simulink model "model"  (R2023b)
settings: Solver=VariableStepAuto  StartTime=0.0  StopTime=10.0  RelTol=1e-3
undefined symbols (not defined in the file): DiscIntNeverNeededParam, Newton, Raphson
libraries: simulink x77, slpidlib x18
(part 1 of 3)
settings Model: Creator=OSCAR4  LastModifiedBy=OSCAR4

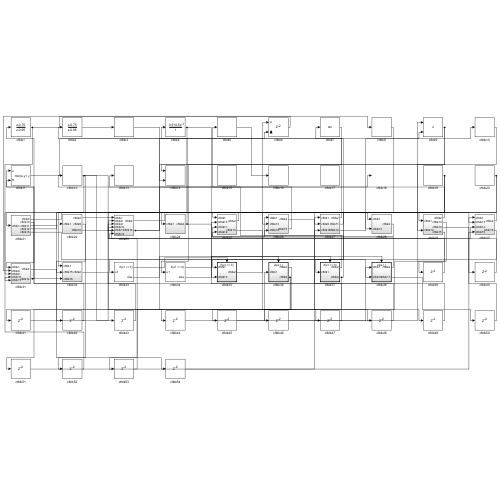
[thumbnail: Simulink's stored preview of the top-level diagram]
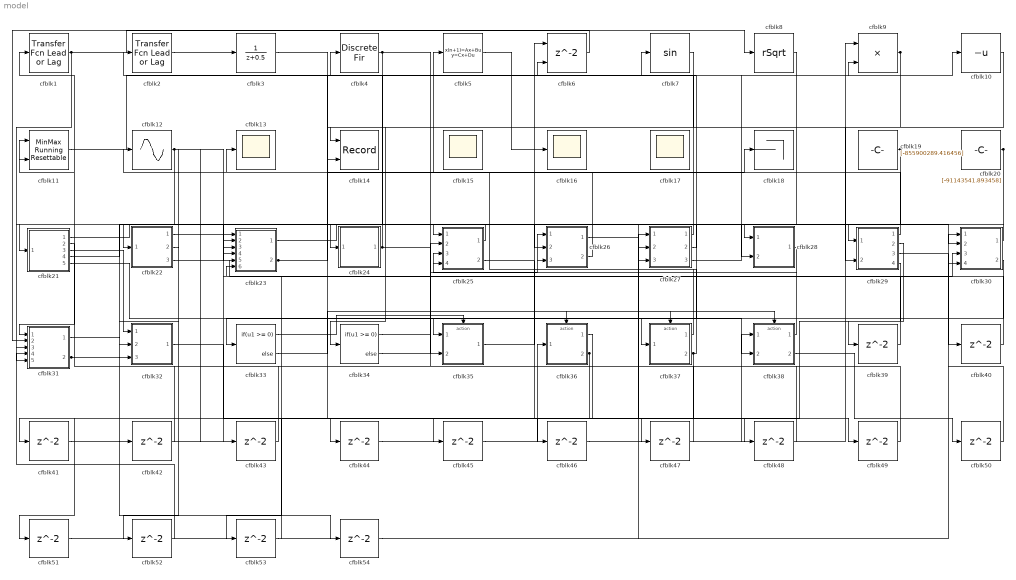
== system model ==
  cfblk1 : simulink/Discrete/Transfer Fcn Lead or Lag  PoleZ=0.95  ZeroZ=0.75  ICPrevOutput=0.0  ICPrevInput=0.0  DoSatur=off
  cfblk10 : UnaryMinus
  cfblk11 : simulink/Math Operations/MinMax Running Resettable  Function=min  vinit=0.0
  cfblk12 : Sin  TimeSource=Use external signal  SampleTime=0
  cfblk{13,15..17} (4 alike) : Scope
      cfblk15 settings: Floating=on
      cfblk17 settings: Floating=on
  cfblk14 : Record  FileSettingsInternal="{\"entries\":[{\"content\":{\"excelSettings\":{\"content\":{},\"type\":\"Streamout.ExcelSettings\"}},\"type\":\"Streamout.FileSettingStorage\",\"uuid\":\"\"}],\"packageUris\":[\"http:\\/\\/schema.mathworks.com\\/mf0\\/streamout_blocks\\/R2020a\"],\"version\":\"1.0\"}"  Layout=[1 1]  SignalsInternal="{\"entries\":[{\"content\":{\"signals\":[{\"content\":{\"blockPath\":[],\"dimensions\":[1],\"domain\":\"\",\"lineColor\":\"#a2142f\",\"plots\":[1],\"port\":1,\"signalID\":8231,\"signalName\":\"XY Graph:1\"},\"type\":\"RecordBlkView.Signal\",\"uuid\":\"\"},{\"content\":{\"blockPath\":[],\"dimensions\":[1],\"domain\":\"\",\"lineColor\":\"#139fff\",\"plots\":[1],\"port\":2,\"signalID\":8234,\"signalName\":\"XY Graph:2\"},\"type\":\"RecordBlkView.Signal\",\"uuid\":\"\"}]},\"type\":\"RecordBlkView.InputSignals\",\"uuid\":\"\"}],\"packageUris\":[\"http:\\/\\/schema.mathworks.com\\/mf0\\/streamout_blocks\\/R2020a\"],\"version\":\"1.0\"}"  VisualizationBindings="{\"xyplotplugin\":{\"info\":[{\"series\":[{\"bindingParametersList\":[{\"parameter\":\"X-Axis\",\"signalID\":8231,\"signalName\":\"XY Graph:1\"},{\"parameter\":\"Y-Axis\",\"signalID\":8234,\"signalName\":\"XY Graph:2\"}],\"seriesID\":32873}],\"subplotID\":1}]}}"  CompatibilityTag=XY
  cfblk18 : Terminator
  cfblk19 : Constant  Value=[-855900289.416456]  SampleTime=1
  cfblk2 : simulink/Discrete/Transfer Fcn Lead or Lag  PoleZ=0.95  ZeroZ=0.75  ICPrevOutput=0.0  ICPrevInput=0.0  DoSatur=off
  cfblk20 : Constant  Value=[-91143541.893458]  SampleTime=1
  cfblk21 : Subsystem
  cfblk22 : Subsystem
  cfblk23 : Subsystem
  cfblk24 : Subsystem
  cfblk25 : Subsystem
  cfblk26 : Subsystem
  cfblk27 : Subsystem
  cfblk28 : Subsystem
  cfblk29 : Subsystem
  cfblk3 : DiscreteTransferFcn  SampleTime=1
  cfblk30 : Subsystem
  cfblk31 : Subsystem
  cfblk32 : Subsystem
  cfblk33 : If  IfExpression=u1 >= 0  SampleTime=1
  cfblk34 : If  IfExpression=u1 >= 0  SampleTime=1
  cfblk35 : Subsystem  TreatAsAtomicUnit=on
  cfblk36 : Subsystem  TreatAsAtomicUnit=on
  cfblk37 : Subsystem  TreatAsAtomicUnit=on
  cfblk38 : Subsystem  TreatAsAtomicUnit=on
  cfblk{39..54} (16 alike) : Delay  SampleTime=1
  cfblk4 : DiscreteFir  SampleTime=1
  cfblk5 : DiscreteStateSpace
  cfblk6 : Delay  ShowEnablePort=on  SampleTime=1
      settings: InputPortMap=u0,e6
  cfblk7 : Trigonometry
  cfblk8 : Sqrt  Operator=rSqrt  AlgorithmType=Newton-Raphson
  cfblk9 : Product
  wires:
  cfblk21/1(cfblk2) -> cfblk25/1(cfblk1)
  cfblk21/2(cfblk10) -> cfblk31/1(cfblk1)
  cfblk5/1 -> cfblk16/1
  cfblk27/1(cfblk2) -> cfblk7/1
  cfblk19/1 -> cfblk33/1, cfblk37/1(cfblk1), cfblk35/2(cfblk13)
  cfblk20/1 -> cfblk21/1(cfblk1), cfblk31/3(cfblk9)
  cfblk29/1(cfblk2) -> cfblk5/1
  cfblk7/1 -> cfblk14/1
  cfblk6/1 -> cfblk31/2(cfblk8)
  cfblk31/2(cfblk12) -> cfblk11/1, cfblk54/1
  cfblk9/1 -> cfblk14/2, cfblk34/1
  cfblk2/1 -> cfblk3/1
  cfblk25/1(cfblk2) -> cfblk24/1(cfblk1)
  cfblk1/1 -> cfblk8/1, cfblk31/5(cfblk11)
  cfblk12/1 -> cfblk32/3(cfblk16), cfblk26/2(cfblk13), cfblk43/1, cfblk52/1
  cfblk30/1(cfblk2) -> cfblk29/1(cfblk1)
  cfblk24/1(cfblk2) -> cfblk2/1, cfblk26/3(cfblk14)
  cfblk11/1 -> cfblk9/2
  cfblk38/1(cfblk2) -> cfblk25/3(cfblk11)
  cfblk28/1(cfblk2) -> cfblk25/4(cfblk12)
  cfblk36/2(cfblk9) -> cfblk46/1, cfblk51/1
  cfblk37/1(cfblk2) -> cfblk12/1
  cfblk21/3(cfblk11) -> cfblk32/1(cfblk1)
  cfblk35/1(cfblk2) -> cfblk6/1
  cfblk10/1 -> cfblk29/2(cfblk12)
  cfblk4/1 -> cfblk22/1(cfblk1), cfblk28/2(cfblk13)
  cfblk30/2(cfblk16) -> cfblk35/1(cfblk1)
  cfblk26/2(cfblk15) -> cfblk13/1
  cfblk27/2(cfblk11) -> cfblk4/1
  cfblk37/2(cfblk8) -> cfblk26/1(cfblk1), cfblk53/1
  cfblk23/1(cfblk2) -> cfblk27/2(cfblk9)
  cfblk22/1(cfblk2) -> cfblk30/2(cfblk13)
  cfblk21/4(cfblk12) -> cfblk28/1(cfblk1)
  cfblk23/2(cfblk13) -> cfblk18/1, cfblk6/2
  cfblk21/5(cfblk13) -> cfblk38/2(cfblk16)
  cfblk22/2(cfblk9) -> cfblk32/2(cfblk15)
  cfblk22/3(cfblk10) -> cfblk30/3(cfblk14)
  cfblk27/3(cfblk12) -> cfblk10/1
  cfblk8/1 -> cfblk23/5(cfblk11)
  cfblk33/1 -> cfblk35/Action
  cfblk33/2 -> cfblk36/Action
  cfblk34/1 -> cfblk37/Action
  cfblk34/2 -> cfblk38/Action
  cfblk29/2(cfblk13) -> cfblk39/1
  cfblk39/1 -> cfblk23/1(cfblk1)
  cfblk29/3(cfblk14) -> cfblk40/1
  cfblk40/1 -> cfblk23/2(cfblk8)
  cfblk29/4(cfblk15) -> cfblk41/1
  cfblk41/1 -> cfblk23/4(cfblk10)
  cfblk31/1(cfblk2) -> cfblk42/1
  cfblk42/1 -> cfblk1/1
  cfblk43/1 -> cfblk11/2
  cfblk32/1(cfblk2) -> cfblk44/1
  cfblk44/1 -> cfblk36/1(cfblk1)
  cfblk36/1(cfblk2) -> cfblk45/1
  cfblk45/1 -> cfblk9/1
  cfblk46/1 -> cfblk38/1(cfblk1)
  cfblk3/1 -> cfblk47/1
  cfblk47/1 -> cfblk27/1(cfblk1)
  cfblk26/1(cfblk2) -> cfblk48/1
  cfblk48/1 -> cfblk25/2(cfblk10)
  cfblk25/2(cfblk13) -> cfblk49/1
  cfblk49/1 -> cfblk23/3(cfblk9)
  cfblk38/2(cfblk17) -> cfblk50/1
  cfblk50/1 -> cfblk30/1(cfblk1)
  cfblk51/1 -> cfblk27/3(cfblk10)
  cfblk52/1 -> cfblk31/4(cfblk10)
  cfblk53/1 -> cfblk23/6(cfblk12)
  cfblk54/1 -> cfblk30/4(cfblk15)

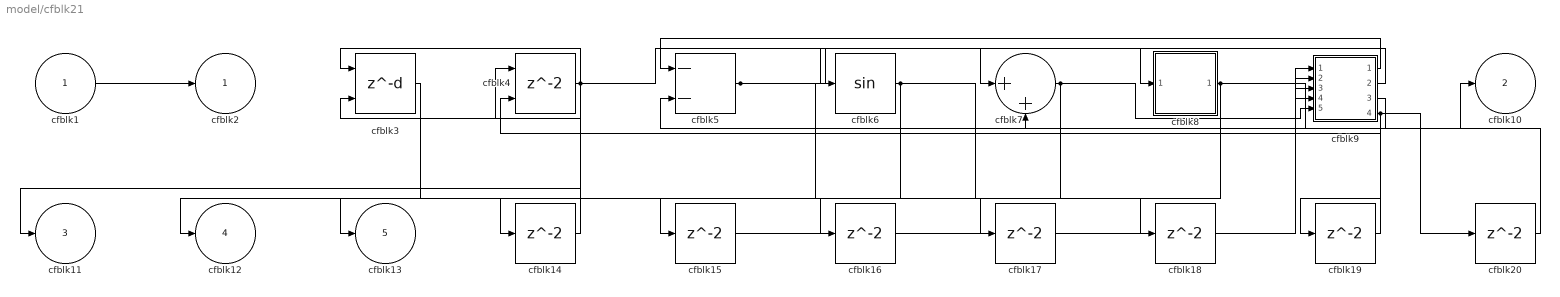
== system model/cfblk21 ==
  cfblk1 : Inport
  cfblk{14..20} (7 alike) : Delay  SampleTime=1
  cfblk3 : Delay  DelayLengthSource=Input port  SampleTime=1
      settings: InputPortMap=u0,p1
  cfblk4 : Delay  ShowEnablePort=on  SampleTime=1
      settings: InputPortMap=u0,e6
  cfblk5 : Sum  Inputs=--
  cfblk6 : Trigonometry
  cfblk7 : Sum  Inputs=|++
  cfblk8 : Subsystem
  cfblk9 : Subsystem
  cfblk2 : Outport
  cfblk10 : Outport  Port=2
  cfblk11 : Outport  Port=3
  cfblk12 : Outport  Port=4
  cfblk13 : Outport  Port=5
  wires:
  cfblk6/1 -> cfblk13/1, cfblk18/1
  cfblk1/1 -> cfblk2/1
  cfblk5/1 -> cfblk8/1(cfblk1), cfblk17/1
  cfblk9/1(cfblk2) -> cfblk5/1
  cfblk4/1 -> cfblk11/1, cfblk3/1, cfblk3/2, cfblk7/1
  cfblk9/2(cfblk15) -> cfblk6/1
  cfblk8/1(cfblk2) -> cfblk10/1, cfblk15/1, cfblk16/1
  cfblk7/1 -> cfblk9/5(cfblk14), cfblk14/1
  cfblk3/1 -> cfblk12/1
  cfblk9/3(cfblk16) -> cfblk5/2
  cfblk9/4(cfblk17) -> cfblk19/1, cfblk20/1
  cfblk14/1 -> cfblk4/1
  cfblk15/1 -> cfblk9/3(cfblk12)
  cfblk16/1 -> cfblk9/4(cfblk13)
  cfblk17/1 -> cfblk9/2(cfblk11)
  cfblk18/1 -> cfblk9/1(cfblk1)
  cfblk19/1 -> cfblk4/2
  cfblk20/1 -> cfblk7/2

== system model/cfblk22 ==
  cfblk1 : Inport
  cfblk{3,11..17} (8 alike) : Delay  SampleTime=1
  cfblk4 : Subsystem
  cfblk5 : Subsystem
  cfblk6 : Subsystem
  cfblk7 : Subsystem
  cfblk8 : Subsystem
  cfblk2 : Outport
  cfblk9 : Outport  Port=2
  cfblk10 : Outport  Port=3
  wires:
  cfblk1/1 -> cfblk8/1(cfblk1)
  cfblk8/1(cfblk2) -> cfblk6/1(cfblk1)
  cfblk4/1(cfblk2) -> cfblk7/1(cfblk1)
  cfblk5/1(cfblk2) -> cfblk3/1
  cfblk3/1 -> cfblk10/1, cfblk4/2(cfblk13), cfblk4/3(cfblk14), cfblk16/1
  cfblk6/1(cfblk2) -> cfblk2/1
  cfblk8/2(cfblk10) -> cfblk5/1(cfblk1)
  cfblk8/3(cfblk11) -> cfblk5/2(cfblk11), cfblk9/1, cfblk4/5(cfblk16)
  cfblk6/2(cfblk9) -> cfblk5/3(cfblk12)
  cfblk5/3(cfblk16) -> cfblk7/2(cfblk9)
  cfblk7/3(cfblk11) -> cfblk13/1, cfblk14/1
  cfblk7/1(cfblk2) -> cfblk11/1
  cfblk11/1 -> cfblk6/4(cfblk8)
  cfblk7/2(cfblk10) -> cfblk12/1
  cfblk12/1 -> cfblk4/1(cfblk1)
  cfblk13/1 -> cfblk5/4(cfblk13)
  cfblk14/1 -> cfblk4/4(cfblk15)
  cfblk4/2(cfblk17) -> cfblk15/1
  cfblk15/1 -> cfblk6/2(cfblk6)
  cfblk16/1 -> cfblk5/5(cfblk14)
  cfblk5/2(cfblk15) -> cfblk17/1
  cfblk17/1 -> cfblk6/3(cfblk7)

== system model/cfblk23 ==
  cfblk1 : Inport
  cfblk8 : Inport  Port=2
  cfblk9 : Inport  Port=3
  cfblk10 : Inport  Port=4
  cfblk11 : Inport  Port=5
  cfblk12 : Inport  Port=6
  cfblk14 : Delay  SampleTime=1
  cfblk15 : Delay  SampleTime=1
  cfblk3 : Delay  ShowEnablePort=on  SampleTime=1
      settings: InputPortMap=u0,e6
  cfblk4 : DotProduct  OutDataTypeStr=Inherit: Inherit via internal rule
  cfblk5 : Subsystem
  cfblk6 : Subsystem
  cfblk7 : Subsystem
  cfblk2 : Outport
  cfblk13 : Outport  Port=2
  wires:
  cfblk4/1 -> cfblk7/1(cfblk1)
  cfblk8/1 -> cfblk5/1(cfblk1)
  cfblk6/2(cfblk10) -> cfblk5/2(cfblk6)
  cfblk12/1 -> cfblk3/2
  cfblk9/1 -> cfblk6/1(cfblk1)
  cfblk3/1 -> cfblk6/2(cfblk8)
  cfblk11/1 -> cfblk4/1
  cfblk7/1(cfblk2) -> cfblk6/3(cfblk9)
  cfblk7/2(cfblk13) -> cfblk2/1, cfblk15/1
  cfblk1/1 -> cfblk5/3(cfblk7)
  cfblk10/1 -> cfblk5/4(cfblk8)
  cfblk5/1(cfblk2) -> cfblk13/1
  cfblk6/1(cfblk2) -> cfblk14/1
  cfblk14/1 -> cfblk3/1
  cfblk15/1 -> cfblk4/2

== system model/cfblk24 ==
  cfblk1 : Inport
  cfblk10 : Delay  SampleTime=1
  cfblk3 : DiscreteFilter  SampleTime=1
  cfblk4 : DiscreteFir  SampleTime=1
  cfblk5 : DiscreteZeroPole  Poles=[0 0.5]  Gain=1
  cfblk6 : Delay  SampleTime=1
  cfblk7 : Constant  Value=[-62407145.955087]  SampleTime=1
  cfblk8 : Constant  Value=[-969597056.657864]  SampleTime=1
  cfblk9 : Constant  Value=[861290801.323652]  SampleTime=1
  cfblk2 : Outport
  wires:
  cfblk7/1 -> cfblk5/1
  cfblk1/1 -> cfblk3/1
  cfblk4/1 -> cfblk6/1
  cfblk5/1 -> cfblk2/1
  cfblk6/1 -> cfblk10/1
  cfblk10/1 -> cfblk4/1

== system model/cfblk25 ==
  cfblk1 : Inport
  cfblk10 : Inport  Port=2
  cfblk11 : Inport  Port=3
  cfblk12 : Inport  Port=4
  cfblk3 : DiscreteFir  SampleTime=1
  cfblk4 : simulink/Discrete/Difference  ICPrevInput=0.0  OutMin=[]  OutMax=[]  OutDataTypeStr=Inherit: Inherit via back propagation  OutDataType=fixdt(1, 16)  OutScaling=2^-10  DoSatur=off
  cfblk5 : Product
  cfblk6 : Sqrt
  cfblk7 : Constant  Value=[-116065568.757723]  SampleTime=1
  cfblk8 : Constant  Value=[768182998.999454]  SampleTime=1
  cfblk9 : Subsystem
  cfblk2 : Outport
  cfblk13 : Outport  Port=2
  wires:
  cfblk1/1 -> cfblk4/1
  cfblk8/1 -> cfblk3/1
  cfblk11/1 -> cfblk2/1
  cfblk10/1 -> cfblk9/1(cfblk1)
  cfblk7/1 -> cfblk13/1
  cfblk5/1 -> cfblk9/2(cfblk5)
  cfblk12/1 -> cfblk6/1
  cfblk6/1 -> cfblk5/1
  cfblk3/1 -> cfblk9/3(cfblk6)
  cfblk4/1 -> cfblk5/2

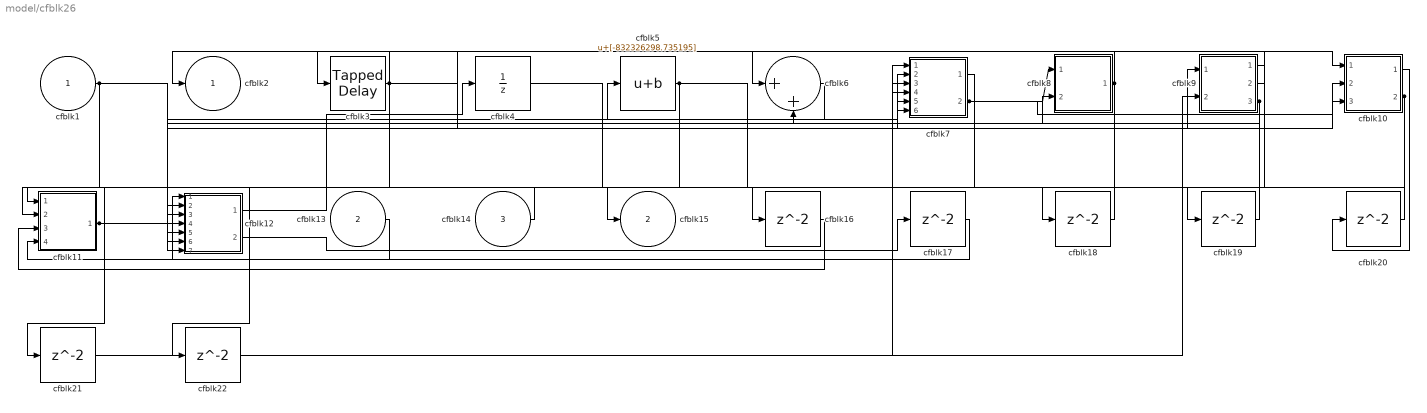
== system model/cfblk26 ==
  cfblk1 : Inport
  cfblk13 : Inport  Port=2
  cfblk14 : Inport  Port=3
  cfblk10 : Subsystem
  cfblk11 : Subsystem
  cfblk12 : Subsystem
  cfblk{16..22} (7 alike) : Delay  SampleTime=1
  cfblk3 : simulink/Discrete/Tapped Delay  vinit=0.0  samptime=-1  NumDelays=1  DelayOrder=Oldest  includeCurrent=off
  cfblk4 : UnitDelay  HasFrameUpgradeWarning=on
  cfblk5 : Bias  Bias=[-832326298.735195]  SaturateOnIntegerOverflow=off
  cfblk6 : Sum  Inputs=|++
  cfblk7 : Subsystem
  cfblk8 : Subsystem
  cfblk9 : Subsystem
  cfblk2 : Outport
  cfblk15 : Outport  Port=2
  wires:
  cfblk5/1 -> cfblk12/5(cfblk13), cfblk19/1
  cfblk1/1 -> cfblk11/1(cfblk1), cfblk7/6(cfblk11)
  cfblk9/1(cfblk2) -> cfblk15/1
  cfblk12/1(cfblk2) -> cfblk4/1
  cfblk13/1 -> cfblk12/1(cfblk1)
  cfblk6/1 -> cfblk5/1
  cfblk3/1 -> cfblk2/1, cfblk8/2(cfblk8), cfblk10/1(cfblk1), cfblk10/3(cfblk11), cfblk22/1
  cfblk14/1 -> cfblk12/2(cfblk10)
  cfblk9/2(cfblk13) -> cfblk3/1
  cfblk9/3(cfblk14) -> cfblk7/2(cfblk7), cfblk12/6(cfblk14)
  cfblk7/1(cfblk2) -> cfblk12/3(cfblk11)
  cfblk8/1(cfblk2) -> cfblk6/1, cfblk18/1
  cfblk10/2(cfblk12) -> cfblk12/4(cfblk12), cfblk12/7(cfblk15), cfblk21/1
  cfblk11/1(cfblk2) -> cfblk7/5(cfblk10), cfblk6/2, cfblk9/1(cfblk1)
  cfblk7/2(cfblk12) -> cfblk8/1(cfblk1), cfblk10/2(cfblk10)
  cfblk4/1 -> cfblk16/1
  cfblk16/1 -> cfblk11/3(cfblk9)
  cfblk12/2(cfblk16) -> cfblk17/1
  cfblk17/1 -> cfblk11/4(cfblk10)
  cfblk18/1 -> cfblk7/3(cfblk8)
  cfblk19/1 -> cfblk7/1(cfblk1)
  cfblk10/1(cfblk2) -> cfblk20/1
  cfblk20/1 -> cfblk11/2(cfblk8)
  cfblk21/1 -> cfblk7/4(cfblk9)
  cfblk22/1 -> cfblk9/2(cfblk12)

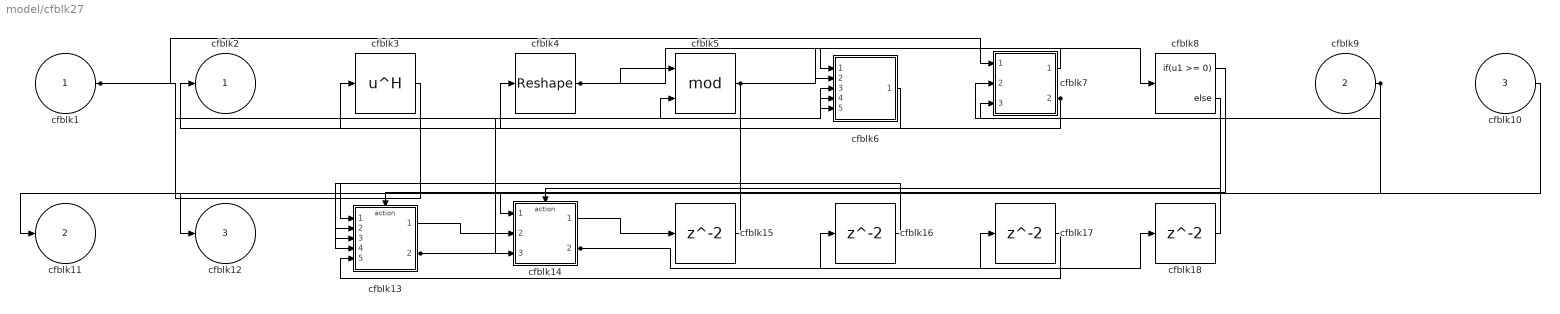
== system model/cfblk27 ==
  cfblk1 : Inport
  cfblk9 : Inport  Port=2
  cfblk10 : Inport  Port=3
  cfblk13 : Subsystem  TreatAsAtomicUnit=on
  cfblk14 : Subsystem  TreatAsAtomicUnit=on
  cfblk{15..18} (4 alike) : Delay  SampleTime=1
  cfblk3 : Math  Operator=hermitian
  cfblk4 : Reshape
  cfblk5 : Math  Operator=mod
  cfblk6 : Subsystem
  cfblk7 : Subsystem
  cfblk8 : If  IfExpression=u1 >= 0  SampleTime=1
  cfblk2 : Outport
  cfblk11 : Outport  Port=2
  cfblk12 : Outport  Port=3
  wires:
  cfblk4/1 -> cfblk6/1(cfblk1), cfblk5/1
  cfblk10/1 -> cfblk11/1
  cfblk9/1 -> cfblk14/1(cfblk1), cfblk14/3(cfblk14), cfblk7/3(cfblk12)
  cfblk6/1(cfblk2) -> cfblk2/1
  cfblk1/1 -> cfblk7/1(cfblk1), cfblk13/4(cfblk14), cfblk5/2
  cfblk14/2(cfblk15) -> cfblk16/1, cfblk17/1, cfblk18/1
  cfblk3/1 -> cfblk13/3(cfblk13)
  cfblk5/1 -> cfblk12/1, cfblk8/1
  cfblk7/1(cfblk2) -> cfblk6/2(cfblk8)
  cfblk13/1(cfblk2) -> cfblk14/2(cfblk13)
  cfblk7/2(cfblk13) -> cfblk3/1, cfblk4/1
  cfblk13/2(cfblk16) -> cfblk6/3(cfblk9), cfblk6/4(cfblk10), cfblk6/5(cfblk11)
  cfblk8/1 -> cfblk13/Action
  cfblk8/2 -> cfblk14/Action
  cfblk14/1(cfblk2) -> cfblk15/1
  cfblk15/1 -> cfblk13/1(cfblk1)
  cfblk16/1 -> cfblk13/2(cfblk12)
  cfblk17/1 -> cfblk13/5(cfblk15)
  cfblk18/1 -> cfblk7/2(cfblk11)

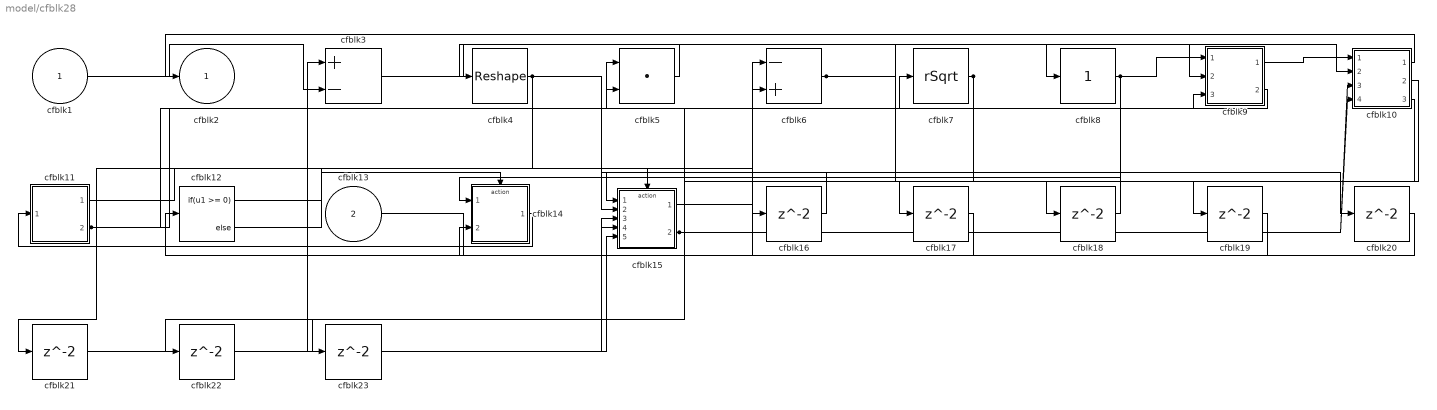
== system model/cfblk28 ==
  cfblk1 : Inport
  cfblk13 : Inport  Port=2
  cfblk10 : Subsystem
  cfblk11 : Subsystem
  cfblk12 : If  IfExpression=u1 >= 0  SampleTime=1
  cfblk14 : Subsystem  TreatAsAtomicUnit=on
  cfblk15 : Subsystem  TreatAsAtomicUnit=on
  cfblk{16..23} (8 alike) : Delay  SampleTime=1
  cfblk3 : Sum  Inputs=+-
  cfblk4 : Reshape
  cfblk5 : DotProduct  OutDataTypeStr=Inherit: Inherit via internal rule
  cfblk6 : Sum  Inputs=-+
  cfblk7 : Sqrt  Operator=rSqrt  AlgorithmType=Newton-Raphson
  cfblk8 : simulink/Math Operations/Slider Gain  gain=1  low=0  high=2
  cfblk9 : Subsystem
  cfblk2 : Outport
  wires:
  cfblk3/1 -> cfblk8/1
  cfblk13/1 -> cfblk6/1
  cfblk15/1(cfblk2) -> cfblk6/2
  cfblk8/1 -> cfblk14/1(cfblk1), cfblk9/1(cfblk1)
  cfblk11/2(cfblk11) -> cfblk7/1, cfblk9/3(cfblk11)
  cfblk7/1 -> cfblk22/1, cfblk23/1
  cfblk14/1(cfblk2) -> cfblk11/1(cfblk1)
  cfblk5/1 -> cfblk4/1
  cfblk9/1(cfblk2) -> cfblk10/1(cfblk1)
  cfblk15/2(cfblk15) -> cfblk5/1, cfblk10/3(cfblk14), cfblk10/4(cfblk15)
  cfblk6/1 -> cfblk10/2(cfblk13), cfblk9/2(cfblk10), cfblk19/1
  cfblk1/1 -> cfblk3/2
  cfblk9/2(cfblk12) -> cfblk5/2
  cfblk4/1 -> cfblk20/1, cfblk21/1
  cfblk10/1(cfblk2) -> cfblk2/1
  cfblk12/1 -> cfblk14/Action
  cfblk12/2 -> cfblk15/Action
  cfblk11/1(cfblk2) -> cfblk16/1
  cfblk16/1 -> cfblk15/1(cfblk1)
  cfblk10/2(cfblk16) -> cfblk17/1
  cfblk17/1 -> cfblk14/2(cfblk10)
  cfblk10/3(cfblk17) -> cfblk18/1
  cfblk18/1 -> cfblk15/2(cfblk11)
  cfblk19/1 -> cfblk15/4(cfblk13)
  cfblk20/1 -> cfblk12/1
  cfblk21/1 -> cfblk15/5(cfblk14)
  cfblk22/1 -> cfblk3/1
  cfblk23/1 -> cfblk15/3(cfblk12)

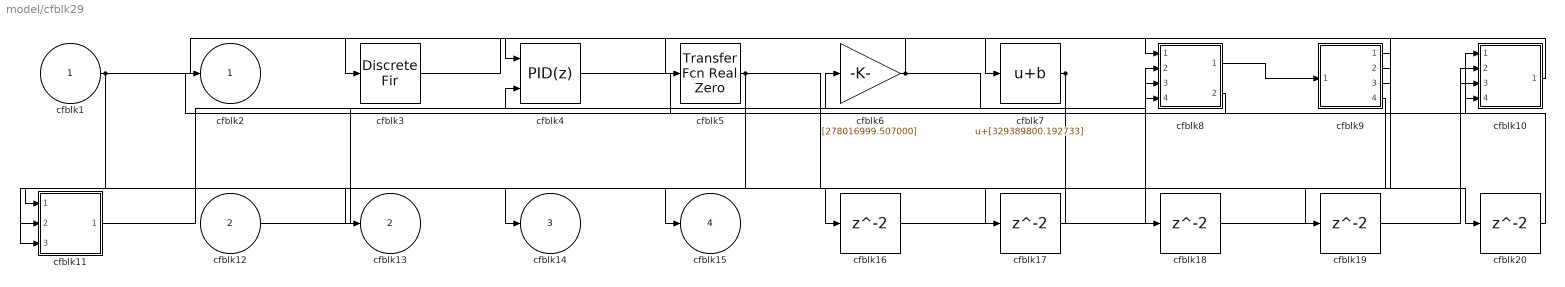
== system model/cfblk29 ==
  cfblk1 : Inport
  cfblk12 : Inport  Port=2
  cfblk10 : Subsystem
  cfblk11 : Subsystem
  cfblk{16..20} (5 alike) : Delay  SampleTime=1
  cfblk3 : DiscreteFir  SampleTime=1
  cfblk4 : slpidlib/PID Controller (2DOF)  Controller=PID  Form=Parallel  TimeDomain=Discrete-time  UseExternalTs=off  SampleTime=1  IntegratorMethod=Forward Euler  FilterMethod=Forward Euler  ControllerParametersSource=internal  P=1  I=1  UseKiTs=off  D=0  N=100  UseFilter=on  b=1  c=1  TunerSelectOption=Transfer Function Based (PID Tuner App)  InitialConditionSource=internal  InitialConditionForIntegrator=0  InitialConditionForFilter=0  DifferentiatorICPrevScaledInput=0  ExternalReset=none  TrackingMode=off  Kt=1  LimitOutput=off  SatLimitsSource=internal  UpperSaturationLimit=inf  LowerSaturationLimit=-inf  LinearizeAsGain=off  AntiWindupMode=none  Kb=1  LimitIntegrator=off  UpperIntegratorSaturationLimit=inf  LowerIntegratorSaturationLimit=-inf  POutMin=[]  POutMax=[]  IOutMin=[]  IOutMax=[]  DOutMin=[]  DOutMax=[]  NOutMin=[]  NOutMax=[]  bOutMin=[]  bOutMax=[]  cOutMin=[]  cOutMax=[]  SumOutMin=[]  SumOutMax=[]  SaturationOutMin=[]  SaturationOutMax=[]  PParamMin=[]  PParamMax=[]  IParamMin=[]  IParamMax=[]  DParamMin=[]  DParamMax=[]  NParamMin=[]  NParamMax=[]  bParamMin=[]  bParamMax=[]  cParamMin=[]  cParamMax=[]  KbParamMin=[]  KbParamMax=[]  KtParamMin=[]  KtParamMax=[]  KbOutMin=[]  KbOutMax=[]  KtOutMin=[]  KtOutMax=[]  IntegratorOutMin=[]  IntegratorOutMax=[]  FilterOutMin=[]  FilterOutMax=[]  SumI1OutMin=[]  SumI1OutMax=[]  SumI2OutMin=[]  SumI2OutMax=[]  SumI3OutMin=[]  SumI3OutMax=[]  SumI4OutMin=[]  SumI4OutMax=[]  SumDOutMin=[]  SumDOutMax=[]  Sum1OutMin=[]  Sum1OutMax=[]  Sum2OutMin=[]  Sum2OutMax=[]  Sum3OutMin=[]  Sum3OutMax=[]  DifferentiatorOutMin=[]  DifferentiatorOutMax=[]  FilterDiffOutCoefMin=[]  FilterDiffOutCoefMax=[]  ReciprocalOutMin=[]  ReciprocalOutMax=[]  SumDenOutMin=[]  SumDenOutMax=[]  SumNumOutMin=[]  SumNumOutMax=[]  DivideOutMin=[]  DivideOutMax=[]  UdiffTsProdOutMin=[]  UdiffTsProdOutMax=[]  NTsProdOutMin=[]  NTsProdOutMax=[]  UintegralTsProdOutMin=[]  UintegralTsProdOutMax=[]  UngainTsProdOutMin=[]  UngainTsProdOutMax=[]  ClampingZeroOutDataTypeStr=Inherit: Inherit via back propagation  ClampingZeroOutMin=[]  ClampingZeroOutMax=[]  FilterDenConstantOutDataTypeStr=Inherit: Inherit via back propagation  FilterDenConstantOutMin=[]  FilterDenConstantOutMax=[]  PCopyOutDataTypeStr=Inherit: Inherit via back propagation  PCopyOutMin=[]  PCopyOutMax=[]  NCopyOutDataTypeStr=Inherit: Inherit via back propagation  NCopyOutMin=[]  NCopyOutMax=[]  IntegratorContinuousStateAttributes=''  IntegratorStateMustResolveToSignalObject=off  IntegratorRTWStateStorageClass=Auto  FilterContinuousStateAttributes=''  FilterStateMustResolveToSignalObject=off  FilterRTWStateStorageClass=Auto  ParallelPVariant=InternalParameters  IdealPVariant=Disabled  IVariant=InternalParameters  DVariant=InternalParameters  bVariant=InternalParameters  cVariant=InternalParameters  IntegratorVariant=Discrete  SatVariant=Disabled  AWVariant=Passthrough  PCopyVariant=Disabled  TRVariant=Disabled  FdbkBlocksVariant=Forward  IdealPFdbkVariant=Disabled  SatFdbkVariant=Disabled  DerivativeFilterVariant=ForwardEulerFilter  NVariant=InternalParameters  NCopyVariant=Disabled  FilterICVariant=InternalICsFilter  IntegratorICVariant=InternalICs  ExternalResetVariant=Disabled  TRSumVariant=Passthrough  SumFdbkVariant=Disabled  SumVariant=Sum_PID  TsampFilterVariant=InternalTs  TsampNgainVariant=Passthrough  TsampIntegralVariant=Disabled_SignalSpec  ExternalSaturationOutDataTypeStr=Inherit: Same as second input
      settings: LibrarySourceBlock=simulink/Discrete/Discrete PID Controller (2DOF)
  cfblk5 : simulink/Discrete/Transfer Fcn Real Zero  ZeroZ=0.75  ICPrevInput=0.0  DoSatur=off
  cfblk6 : Gain  Gain=[278016999.507000]
  cfblk7 : Bias  Bias=[329389800.192733]  SaturateOnIntegerOverflow=off
  cfblk8 : Subsystem
  cfblk9 : Subsystem
  cfblk2 : Outport
  cfblk13 : Outport  Port=2
  cfblk14 : Outport  Port=3
  cfblk15 : Outport  Port=4
  wires:
  cfblk6/1 -> cfblk3/1, cfblk8/3(cfblk14)
  cfblk4/1 -> cfblk10/1(cfblk1)
  cfblk12/1 -> cfblk6/1
  cfblk10/1(cfblk2) -> cfblk5/1
  cfblk1/1 -> cfblk4/1, cfblk11/3(cfblk8)
  cfblk5/1 -> cfblk11/1(cfblk1), cfblk13/1, cfblk11/2(cfblk7), cfblk19/1, cfblk20/1
  cfblk8/1(cfblk2) -> cfblk9/1(cfblk1)
  cfblk8/2(cfblk16) -> cfblk2/1
  cfblk3/1 -> cfblk8/1(cfblk1)
  cfblk9/1(cfblk2) -> cfblk14/1
  cfblk11/1(cfblk2) -> cfblk8/2(cfblk13)
  cfblk9/2(cfblk12) -> cfblk7/1
  cfblk7/1 -> cfblk15/1, cfblk16/1
  cfblk16/1 -> cfblk8/4(cfblk15)
  cfblk9/3(cfblk13) -> cfblk17/1
  cfblk17/1 -> cfblk4/2
  cfblk9/4(cfblk14) -> cfblk18/1
  cfblk18/1 -> cfblk10/2(cfblk14)
  cfblk19/1 -> cfblk10/3(cfblk15)
  cfblk20/1 -> cfblk10/4(cfblk16)

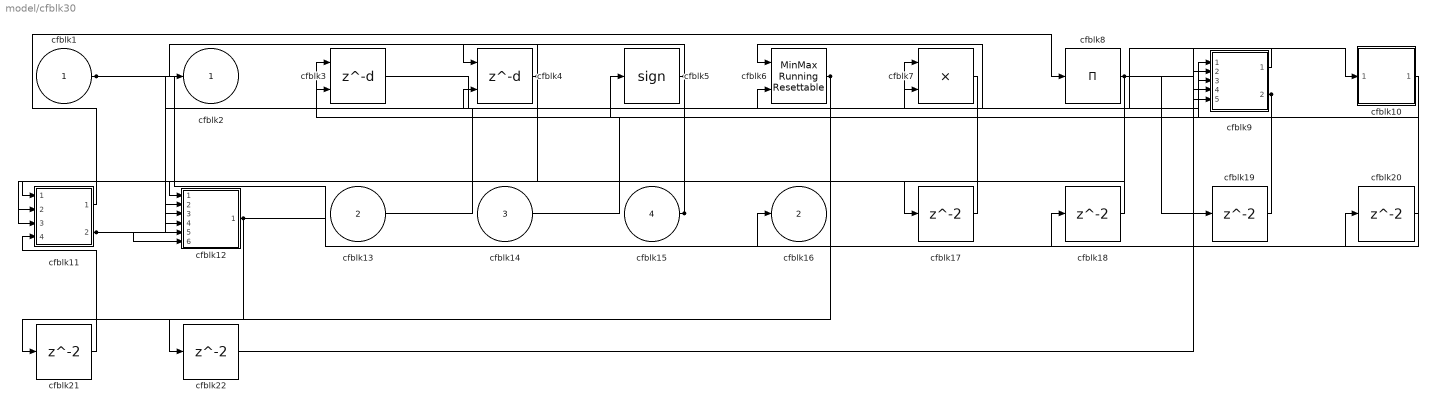
== system model/cfblk30 ==
  cfblk1 : Inport
  cfblk13 : Inport  Port=2
  cfblk14 : Inport  Port=3
  cfblk15 : Inport  Port=4
  cfblk10 : Subsystem
  cfblk11 : Subsystem
  cfblk12 : Subsystem
  cfblk{17..22} (6 alike) : Delay  SampleTime=1
  cfblk3 : Delay  DelayLengthSource=Input port  SampleTime=1
      settings: InputPortMap=u0,p1
  cfblk4 : Delay  DelayLengthSource=Input port  SampleTime=1
      settings: InputPortMap=u0,p1
  cfblk5 : Signum
  cfblk6 : simulink/Math Operations/MinMax Running Resettable  Function=min  vinit=0.0
  cfblk7 : Product
  cfblk8 : Product  Inputs=*
  cfblk9 : Subsystem
  cfblk2 : Outport
  cfblk16 : Outport  Port=2
  wires:
  cfblk13/1 -> cfblk7/1
  cfblk14/1 -> cfblk9/1(cfblk1)
  cfblk5/1 -> cfblk4/1, cfblk11/3(cfblk10)
  cfblk1/1 -> cfblk16/1, cfblk9/3(cfblk9)
  cfblk11/1(cfblk2) -> cfblk8/1
  cfblk3/1 -> cfblk7/2
  cfblk4/1 -> cfblk2/1, cfblk12/4(cfblk13)
  cfblk9/1(cfblk2) -> cfblk6/1
  cfblk15/1 -> cfblk12/1(cfblk1), cfblk12/3(cfblk12)
  cfblk11/2(cfblk12) -> cfblk4/2, cfblk3/1, cfblk12/6(cfblk15)
  cfblk9/2(cfblk12) -> cfblk5/1, cfblk3/2
  cfblk7/1 -> cfblk12/2(cfblk11)
  cfblk8/1 -> cfblk10/1(cfblk1), cfblk12/5(cfblk14), cfblk17/1, cfblk19/1
  cfblk12/1(cfblk2) -> cfblk20/1, cfblk21/1
  cfblk6/1 -> cfblk11/2(cfblk9), cfblk22/1
  cfblk17/1 -> cfblk6/2
  cfblk10/1(cfblk2) -> cfblk18/1
  cfblk18/1 -> cfblk11/1(cfblk1)
  cfblk19/1 -> cfblk9/4(cfblk10)
  cfblk20/1 -> cfblk9/2(cfblk8)
  cfblk21/1 -> cfblk11/4(cfblk11)
  cfblk22/1 -> cfblk9/5(cfblk11)

== system model/cfblk31 ==
  cfblk1 : Inport
  cfblk8 : Inport  Port=2
  cfblk9 : Inport  Port=3
  cfblk10 : Inport  Port=4
  cfblk11 : Inport  Port=5
  cfblk13 : Delay  SampleTime=1
  cfblk3 : DiscreteFilter  SampleTime=1
  cfblk4 : Sum
  cfblk5 : Subsystem
  cfblk6 : Subsystem
  cfblk7 : Subsystem
  cfblk2 : Outport
  cfblk12 : Outport  Port=2
  wires:
  cfblk4/1 -> cfblk6/1(cfblk1)
  cfblk9/1 -> cfblk7/1(cfblk1), cfblk6/3(cfblk7)
  cfblk8/1 -> cfblk7/2(cfblk10)
  cfblk1/1 -> cfblk5/1(cfblk1)
  cfblk6/1(cfblk2) -> cfblk7/3(cfblk11)
  cfblk11/1 -> cfblk5/2(cfblk8)
  cfblk5/1(cfblk2) -> cfblk4/2
  cfblk10/1 -> cfblk6/2(cfblk6)
  cfblk3/1 -> cfblk12/1
  cfblk5/2(cfblk9) -> cfblk3/1
  cfblk5/3(cfblk10) -> cfblk2/1
  cfblk7/1(cfblk2) -> cfblk13/1
  cfblk13/1 -> cfblk4/1

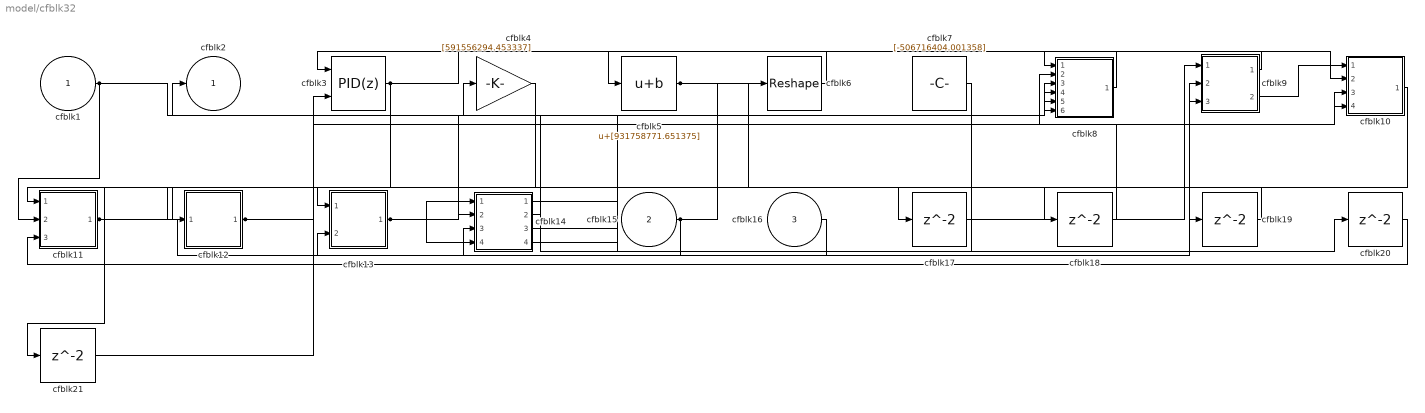
== system model/cfblk32 ==
  cfblk1 : Inport
  cfblk15 : Inport  Port=2
  cfblk16 : Inport  Port=3
  cfblk10 : Subsystem
  cfblk11 : Subsystem
  cfblk12 : Subsystem
  cfblk13 : Subsystem
  cfblk14 : Subsystem
  cfblk{17..21} (5 alike) : Delay  SampleTime=1
  cfblk3 : slpidlib/PID Controller (2DOF)  Controller=PID  Form=Parallel  TimeDomain=Discrete-time  UseExternalTs=off  SampleTime=1  IntegratorMethod=Forward Euler  FilterMethod=Forward Euler  ControllerParametersSource=internal  P=1  I=1  UseKiTs=off  D=0  N=100  UseFilter=on  b=1  c=1  TunerSelectOption=Transfer Function Based (PID Tuner App)  InitialConditionSource=internal  InitialConditionForIntegrator=0  InitialConditionForFilter=0  DifferentiatorICPrevScaledInput=0  ExternalReset=none  TrackingMode=off  Kt=1  LimitOutput=off  SatLimitsSource=internal  UpperSaturationLimit=inf  LowerSaturationLimit=-inf  LinearizeAsGain=off  AntiWindupMode=none  Kb=1  LimitIntegrator=off  UpperIntegratorSaturationLimit=inf  LowerIntegratorSaturationLimit=-inf  POutMin=[]  POutMax=[]  IOutMin=[]  IOutMax=[]  DOutMin=[]  DOutMax=[]  NOutMin=[]  NOutMax=[]  bOutMin=[]  bOutMax=[]  cOutMin=[]  cOutMax=[]  SumOutMin=[]  SumOutMax=[]  SaturationOutMin=[]  SaturationOutMax=[]  PParamMin=[]  PParamMax=[]  IParamMin=[]  IParamMax=[]  DParamMin=[]  DParamMax=[]  NParamMin=[]  NParamMax=[]  bParamMin=[]  bParamMax=[]  cParamMin=[]  cParamMax=[]  KbParamMin=[]  KbParamMax=[]  KtParamMin=[]  KtParamMax=[]  KbOutMin=[]  KbOutMax=[]  KtOutMin=[]  KtOutMax=[]  IntegratorOutMin=[]  IntegratorOutMax=[]  FilterOutMin=[]  FilterOutMax=[]  SumI1OutMin=[]  SumI1OutMax=[]  SumI2OutMin=[]  SumI2OutMax=[]  SumI3OutMin=[]  SumI3OutMax=[]  SumI4OutMin=[]  SumI4OutMax=[]  SumDOutMin=[]  SumDOutMax=[]  Sum1OutMin=[]  Sum1OutMax=[]  Sum2OutMin=[]  Sum2OutMax=[]  Sum3OutMin=[]  Sum3OutMax=[]  DifferentiatorOutMin=[]  DifferentiatorOutMax=[]  FilterDiffOutCoefMin=[]  FilterDiffOutCoefMax=[]  ReciprocalOutMin=[]  ReciprocalOutMax=[]  SumDenOutMin=[]  SumDenOutMax=[]  SumNumOutMin=[]  SumNumOutMax=[]  DivideOutMin=[]  DivideOutMax=[]  UdiffTsProdOutMin=[]  UdiffTsProdOutMax=[]  NTsProdOutMin=[]  NTsProdOutMax=[]  UintegralTsProdOutMin=[]  UintegralTsProdOutMax=[]  UngainTsProdOutMin=[]  UngainTsProdOutMax=[]  ClampingZeroOutDataTypeStr=Inherit: Inherit via back propagation  ClampingZeroOutMin=[]  ClampingZeroOutMax=[]  FilterDenConstantOutDataTypeStr=Inherit: Inherit via back propagation  FilterDenConstantOutMin=[]  FilterDenConstantOutMax=[]  PCopyOutDataTypeStr=Inherit: Inherit via back propagation  PCopyOutMin=[]  PCopyOutMax=[]  NCopyOutDataTypeStr=Inherit: Inherit via back propagation  NCopyOutMin=[]  NCopyOutMax=[]  IntegratorContinuousStateAttributes=''  IntegratorStateMustResolveToSignalObject=off  IntegratorRTWStateStorageClass=Auto  FilterContinuousStateAttributes=''  FilterStateMustResolveToSignalObject=off  FilterRTWStateStorageClass=Auto  ParallelPVariant=InternalParameters  IdealPVariant=Disabled  IVariant=InternalParameters  DVariant=InternalParameters  bVariant=InternalParameters  cVariant=InternalParameters  IntegratorVariant=Discrete  SatVariant=Disabled  AWVariant=Passthrough  PCopyVariant=Disabled  TRVariant=Disabled  FdbkBlocksVariant=Forward  IdealPFdbkVariant=Disabled  SatFdbkVariant=Disabled  DerivativeFilterVariant=ForwardEulerFilter  NVariant=InternalParameters  NCopyVariant=Disabled  FilterICVariant=InternalICsFilter  IntegratorICVariant=InternalICs  ExternalResetVariant=Disabled  TRSumVariant=Passthrough  SumFdbkVariant=Disabled  SumVariant=Sum_PID  TsampFilterVariant=InternalTs  TsampNgainVariant=Passthrough  TsampIntegralVariant=Disabled_SignalSpec  ExternalSaturationOutDataTypeStr=Inherit: Same as second input
      settings: LibrarySourceBlock=simulink/Discrete/Discrete PID Controller (2DOF)
  cfblk4 : Gain  Gain=[591556294.453337]
  cfblk5 : Bias  Bias=[931758771.651375]  SaturateOnIntegerOverflow=off
  cfblk6 : Reshape
  cfblk7 : Constant  Value=[-506716404.001358]  SampleTime=1
  cfblk8 : Subsystem
  cfblk9 : Subsystem
  cfblk2 : Outport
  wires:
  cfblk6/1 -> cfblk3/1
  cfblk15/1 -> cfblk6/1, cfblk14/3(cfblk10)
  cfblk5/1 -> cfblk10/4(cfblk8), cfblk17/1
  cfblk11/1(cfblk2) -> cfblk9/2(cfblk5), cfblk14/2(cfblk9)
  cfblk7/1 -> cfblk13/1(cfblk1)
  cfblk16/1 -> cfblk13/2(cfblk8)
  cfblk13/1(cfblk2) -> cfblk14/1(cfblk1), cfblk8/4(cfblk12), cfblk14/4(cfblk11), cfblk10/3(cfblk7)
  cfblk3/1 -> cfblk12/1(cfblk1), cfblk10/2(cfblk6)
  cfblk1/1 -> cfblk11/2(cfblk13), cfblk8/5(cfblk13), cfblk8/6(cfblk14)
  cfblk12/1(cfblk2) -> cfblk9/3(cfblk6), cfblk4/1
  cfblk14/2(cfblk12) -> cfblk2/1
  cfblk9/1(cfblk2) -> cfblk8/1(cfblk1)
  cfblk9/2(cfblk7) -> cfblk10/1(cfblk1)
  cfblk8/1(cfblk2) -> cfblk5/1
  cfblk14/4(cfblk14) -> cfblk8/3(cfblk11)
  cfblk17/1 -> cfblk9/1(cfblk1)
  cfblk10/1(cfblk2) -> cfblk18/1
  cfblk18/1 -> cfblk8/2(cfblk10)
  cfblk14/1(cfblk2) -> cfblk19/1
  cfblk19/1 -> cfblk11/1(cfblk1)
  cfblk14/3(cfblk13) -> cfblk20/1
  cfblk20/1 -> cfblk11/3(cfblk14)
  cfblk4/1 -> cfblk21/1
  cfblk21/1 -> cfblk3/2

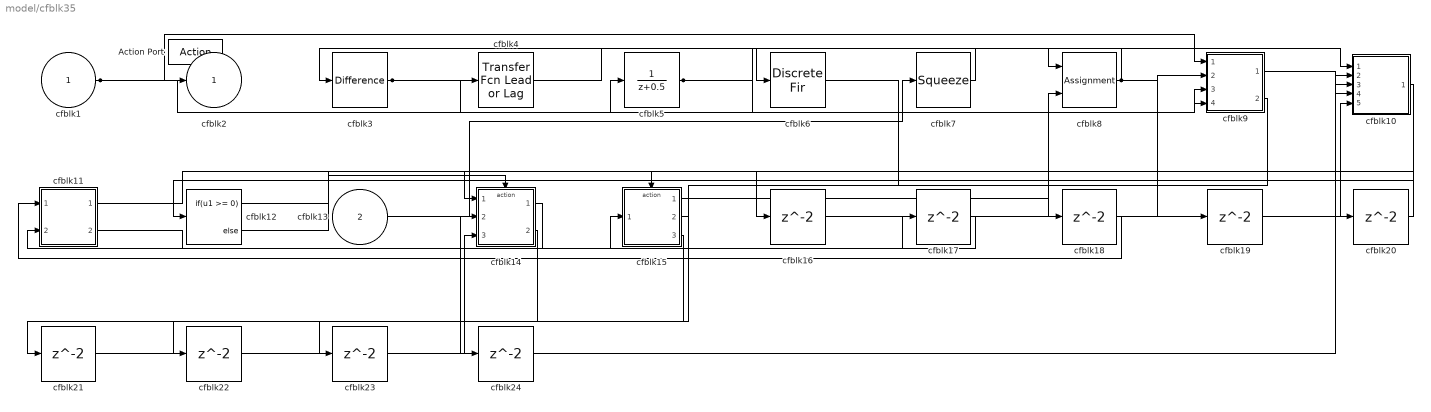
== system model/cfblk35 ==
  cfblk1 : Inport
  cfblk13 : Inport  Port=2
  Action Port : ActionPort  ActionPortLabel=if(u1 >= 0)
  cfblk10 : Subsystem
  cfblk11 : Subsystem
  cfblk12 : If  IfExpression=u1 >= 0  SampleTime=1
  cfblk14 : Subsystem  TreatAsAtomicUnit=on
  cfblk15 : Subsystem  TreatAsAtomicUnit=on
  cfblk{16..24} (9 alike) : Delay
  cfblk3 : simulink/Discrete/Difference  ICPrevInput=0.0  OutMin=[]  OutMax=[]  OutDataTypeStr=Inherit: Inherit via back propagation  OutDataType=fixdt(1, 16)  OutScaling=2^-10  DoSatur=off
  cfblk4 : simulink/Discrete/Transfer Fcn Lead or Lag  PoleZ=0.95  ZeroZ=0.75  ICPrevOutput=0.0  ICPrevInput=0.0  DoSatur=off
  cfblk5 : DiscreteTransferFcn
  cfblk6 : DiscreteFir
  cfblk7 : Squeeze
  cfblk8 : Assignment  DiagnosticForDimensions=Warning  IndexOptions=Index vector (dialog)  Indices=1  OutputSizes=1
  cfblk9 : Subsystem
  cfblk2 : Outport
  wires:
  cfblk1/1 -> cfblk5/1, cfblk2/1, cfblk9/1(cfblk1)
  cfblk13/1 -> cfblk7/1
  cfblk4/1 -> cfblk8/1
  cfblk3/1 -> cfblk4/1, cfblk9/3(cfblk9)
  cfblk8/1 -> cfblk6/1, cfblk9/2(cfblk8), cfblk19/1
  cfblk5/1 -> cfblk10/1(cfblk1), cfblk9/4(cfblk10)
  cfblk7/1 -> cfblk3/1
  cfblk14/1(cfblk2) -> cfblk11/2(cfblk12)
  cfblk15/1(cfblk2) -> cfblk8/2
  cfblk10/1(cfblk2) -> cfblk12/1
  cfblk12/1 -> cfblk14/Action
  cfblk12/2 -> cfblk15/Action
  cfblk11/1(cfblk2) -> cfblk16/1
  cfblk16/1 -> cfblk10/2(cfblk10)
  cfblk11/2(cfblk13) -> cfblk17/1
  cfblk17/1 -> cfblk15/1(cfblk1)
  cfblk6/1 -> cfblk18/1
  cfblk18/1 -> cfblk11/1(cfblk1)
  cfblk19/1 -> cfblk10/5(cfblk13)
  cfblk9/1(cfblk2) -> cfblk20/1
  cfblk20/1 -> cfblk14/1(cfblk1)
  cfblk9/2(cfblk11) -> cfblk21/1
  cfblk21/1 -> cfblk14/2(cfblk5)
  cfblk15/2(cfblk14) -> cfblk22/1
  cfblk22/1 -> cfblk10/4(cfblk12)
  cfblk15/3(cfblk15) -> cfblk23/1
  cfblk23/1 -> cfblk14/3(cfblk6)
  cfblk14/2(cfblk7) -> cfblk24/1
  cfblk24/1 -> cfblk10/3(cfblk11)

== system model/cfblk36 ==
  cfblk1 : Inport
  Action Port : ActionPort  ActionPortLabel=else
  cfblk{3,10..13} (5 alike) : Delay
  cfblk4 : DiscreteIntegrator  SampleTime=-1  ICPrevOutput=DiscIntNeverNeededParam  ICPrevScaledInput=DiscIntNeverNeededParam
  cfblk5 : DotProduct  OutDataTypeStr=Inherit: Inherit via internal rule
  cfblk6 : Subsystem
  cfblk7 : Subsystem
  cfblk8 : Subsystem
  cfblk2 : Outport
  cfblk9 : Outport  Port=2
  wires:
  cfblk4/1 -> cfblk9/1, cfblk8/3(cfblk8), cfblk6/2(cfblk13)
  cfblk5/1 -> cfblk4/1
  cfblk8/1(cfblk2) -> cfblk6/1(cfblk1)
  cfblk6/2(cfblk14) -> cfblk7/1(cfblk1), cfblk2/1
  cfblk1/1 -> cfblk5/1
  cfblk8/2(cfblk9) -> cfblk7/2(cfblk13), cfblk13/1
  cfblk7/2(cfblk15) -> cfblk3/1
  cfblk6/1(cfblk2) -> cfblk10/1
  cfblk10/1 -> cfblk8/1(cfblk1)
  cfblk7/1(cfblk2) -> cfblk11/1
  cfblk11/1 -> cfblk8/2(cfblk7)
  cfblk3/1 -> cfblk12/1
  cfblk12/1 -> cfblk7/3(cfblk14)
  cfblk13/1 -> cfblk5/2

== system model/cfblk37 ==
  cfblk1 : Inport
  Action Port : ActionPort  ActionPortLabel=if(u1 >= 0)
  cfblk{9..16} (8 alike) : Delay
  cfblk3 : Reshape
  cfblk4 : Subsystem
  cfblk5 : Subsystem
  cfblk6 : Subsystem
  cfblk7 : Subsystem
  cfblk2 : Outport
  cfblk8 : Outport  Port=2
  wires:
  cfblk6/1(cfblk2) -> cfblk8/1, cfblk7/4(cfblk7), cfblk5/1(cfblk1)
  cfblk3/1 -> cfblk2/1, cfblk9/1
  cfblk4/1(cfblk2) -> cfblk3/1
  cfblk5/3(cfblk16) -> cfblk14/1, cfblk15/1
  cfblk1/1 -> cfblk6/1(cfblk1)
  cfblk7/1(cfblk2) -> cfblk4/4(cfblk14), cfblk16/1
  cfblk4/3(cfblk16) -> cfblk5/2(cfblk14), cfblk11/1
  cfblk9/1 -> cfblk7/3(cfblk6)
  cfblk4/2(cfblk15) -> cfblk10/1
  cfblk10/1 -> cfblk7/1(cfblk1)
  cfblk11/1 -> cfblk7/2(cfblk5)
  cfblk5/1(cfblk2) -> cfblk12/1
  cfblk12/1 -> cfblk4/1(cfblk1)
  cfblk5/2(cfblk15) -> cfblk13/1
  cfblk13/1 -> cfblk4/2(cfblk12)
  cfblk14/1 -> cfblk4/3(cfblk13)
  cfblk15/1 -> cfblk6/3(cfblk9)
  cfblk16/1 -> cfblk6/2(cfblk8)

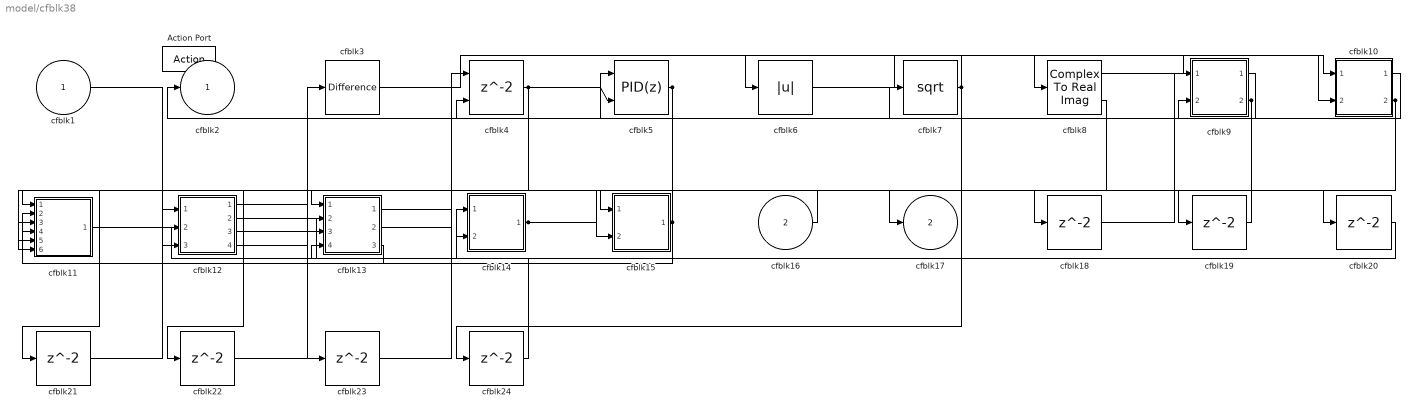
== system model/cfblk38 ==
  cfblk1 : Inport
  cfblk16 : Inport  Port=2
  Action Port : ActionPort  ActionPortLabel=else
  cfblk10 : Subsystem
  cfblk11 : Subsystem
  cfblk12 : Subsystem
  cfblk13 : Subsystem
  cfblk14 : Subsystem
  cfblk15 : Subsystem
  cfblk{18..24} (7 alike) : Delay
  cfblk3 : simulink/Discrete/Difference  ICPrevInput=0.0  OutMin=[]  OutMax=[]  OutDataTypeStr=Inherit: Inherit via back propagation  OutDataType=fixdt(1, 16)  OutScaling=2^-10  DoSatur=off
  cfblk4 : Delay  ShowEnablePort=on
      settings: InputPortMap=u0,e6
  cfblk5 : slpidlib/PID Controller (2DOF)  Controller=PID  Form=Parallel  TimeDomain=Discrete-time  UseExternalTs=off  SampleTime=-1  IntegratorMethod=Forward Euler  FilterMethod=Forward Euler  ControllerParametersSource=internal  P=1  I=1  UseKiTs=off  D=0  N=100  UseFilter=on  b=1  c=1  TunerSelectOption=Transfer Function Based (PID Tuner App)  InitialConditionSource=internal  InitialConditionForIntegrator=0  InitialConditionForFilter=0  DifferentiatorICPrevScaledInput=0  ExternalReset=none  TrackingMode=off  Kt=1  LimitOutput=off  SatLimitsSource=internal  UpperSaturationLimit=inf  LowerSaturationLimit=-inf  LinearizeAsGain=off  AntiWindupMode=none  Kb=1  LimitIntegrator=off  UpperIntegratorSaturationLimit=inf  LowerIntegratorSaturationLimit=-inf  POutMin=[]  POutMax=[]  IOutMin=[]  IOutMax=[]  DOutMin=[]  DOutMax=[]  NOutMin=[]  NOutMax=[]  bOutMin=[]  bOutMax=[]  cOutMin=[]  cOutMax=[]  SumOutMin=[]  SumOutMax=[]  SaturationOutMin=[]  SaturationOutMax=[]  PParamMin=[]  PParamMax=[]  IParamMin=[]  IParamMax=[]  DParamMin=[]  DParamMax=[]  NParamMin=[]  NParamMax=[]  bParamMin=[]  bParamMax=[]  cParamMin=[]  cParamMax=[]  KbParamMin=[]  KbParamMax=[]  KtParamMin=[]  KtParamMax=[]  KbOutMin=[]  KbOutMax=[]  KtOutMin=[]  KtOutMax=[]  IntegratorOutMin=[]  IntegratorOutMax=[]  FilterOutMin=[]  FilterOutMax=[]  SumI1OutMin=[]  SumI1OutMax=[]  SumI2OutMin=[]  SumI2OutMax=[]  SumI3OutMin=[]  SumI3OutMax=[]  SumI4OutMin=[]  SumI4OutMax=[]  SumDOutMin=[]  SumDOutMax=[]  Sum1OutMin=[]  Sum1OutMax=[]  Sum2OutMin=[]  Sum2OutMax=[]  Sum3OutMin=[]  Sum3OutMax=[]  DifferentiatorOutMin=[]  DifferentiatorOutMax=[]  FilterDiffOutCoefMin=[]  FilterDiffOutCoefMax=[]  ReciprocalOutMin=[]  ReciprocalOutMax=[]  SumDenOutMin=[]  SumDenOutMax=[]  SumNumOutMin=[]  SumNumOutMax=[]  DivideOutMin=[]  DivideOutMax=[]  UdiffTsProdOutMin=[]  UdiffTsProdOutMax=[]  NTsProdOutMin=[]  NTsProdOutMax=[]  UintegralTsProdOutMin=[]  UintegralTsProdOutMax=[]  UngainTsProdOutMin=[]  UngainTsProdOutMax=[]  ClampingZeroOutDataTypeStr=Inherit: Inherit via back propagation  ClampingZeroOutMin=[]  ClampingZeroOutMax=[]  FilterDenConstantOutDataTypeStr=Inherit: Inherit via back propagation  FilterDenConstantOutMin=[]  FilterDenConstantOutMax=[]  PCopyOutDataTypeStr=Inherit: Inherit via back propagation  PCopyOutMin=[]  PCopyOutMax=[]  NCopyOutDataTypeStr=Inherit: Inherit via back propagation  NCopyOutMin=[]  NCopyOutMax=[]  IntegratorContinuousStateAttributes=''  IntegratorStateMustResolveToSignalObject=off  IntegratorRTWStateStorageClass=Auto  FilterContinuousStateAttributes=''  FilterStateMustResolveToSignalObject=off  FilterRTWStateStorageClass=Auto  ParallelPVariant=InternalParameters  IdealPVariant=Disabled  IVariant=InternalParameters  DVariant=InternalParameters  bVariant=InternalParameters  cVariant=InternalParameters  IntegratorVariant=Discrete  SatVariant=Disabled  AWVariant=Passthrough  PCopyVariant=Disabled  TRVariant=Disabled  FdbkBlocksVariant=Forward  IdealPFdbkVariant=Disabled  SatFdbkVariant=Disabled  DerivativeFilterVariant=ForwardEulerFilter  NVariant=InternalParameters  NCopyVariant=Disabled  FilterICVariant=InternalICsFilter  IntegratorICVariant=InternalICs  ExternalResetVariant=Disabled  TRSumVariant=Passthrough  SumFdbkVariant=Disabled  SumVariant=Sum_PID  TsampFilterVariant=InternalTs  TsampNgainVariant=Passthrough  TsampIntegralVariant=Disabled_SignalSpec  ExternalSaturationOutDataTypeStr=Inherit: Same as second input
      settings: LibrarySourceBlock=simulink/Discrete/Discrete PID Controller (2DOF)
  cfblk6 : Abs  SaturateOnIntegerOverflow=off
  cfblk7 : Sqrt
  cfblk8 : ComplexToRealImag
  cfblk9 : Subsystem
  cfblk2 : Outport
  cfblk17 : Outport  Port=2
  wires:
  cfblk16/1 -> cfblk11/1(cfblk1)
  cfblk10/1(cfblk2) -> cfblk2/1
  cfblk1/1 -> cfblk13/1(cfblk1)
  cfblk15/1(cfblk2) -> cfblk5/1, cfblk11/4(cfblk11)
  cfblk4/1 -> cfblk5/2, cfblk11/5(cfblk12)
  cfblk6/1 -> cfblk10/1(cfblk1)
  cfblk3/1 -> cfblk8/1
  cfblk8/1 -> cfblk10/2(cfblk8)
  cfblk11/1(cfblk2) -> cfblk14/1(cfblk1)
  cfblk10/2(cfblk9) -> cfblk17/1, cfblk21/1
  cfblk14/1(cfblk2) -> cfblk19/1, cfblk20/1
  cfblk13/1(cfblk2) -> cfblk9/2(cfblk11)
  cfblk7/1 -> cfblk6/1, cfblk15/2(cfblk7), cfblk24/1
  cfblk12/2(cfblk12) -> cfblk14/2(cfblk8)
  cfblk5/1 -> cfblk12/3(cfblk11), cfblk11/3(cfblk10)
  cfblk12/3(cfblk13) -> cfblk3/1
  cfblk9/1(cfblk2) -> cfblk4/2
  cfblk13/2(cfblk16) -> cfblk7/1
  cfblk13/3(cfblk17) -> cfblk11/2(cfblk9)
  cfblk9/2(cfblk12) -> cfblk15/1(cfblk1), cfblk11/6(cfblk13)
  cfblk12/1(cfblk2) -> cfblk18/1
  cfblk18/1 -> cfblk9/1(cfblk1)
  cfblk19/1 -> cfblk12/2(cfblk10)
  cfblk20/1 -> cfblk13/4(cfblk15)
  cfblk21/1 -> cfblk12/1(cfblk1)
  cfblk8/2 -> cfblk22/1
  cfblk22/1 -> cfblk13/2(cfblk13)
  cfblk12/4(cfblk14) -> cfblk23/1
  cfblk23/1 -> cfblk4/1
  cfblk24/1 -> cfblk13/3(cfblk14)

== system model/cfblk21/cfblk8 ==
  cfblk1 : Inport
  cfblk10 : DotProduct  OutDataTypeStr=Inherit: Inherit via internal rule
  cfblk11 : Constant  Value=[-944773892.989427]  SampleTime=1
  cfblk12 : Constant  Value=[686051792.779080]  SampleTime=1
  cfblk13 : Delay  SampleTime=1
  cfblk3 : Delay  ShowEnablePort=on  SampleTime=1
      settings: InputPortMap=u0,e6
  cfblk4 : PropagationDelay  SampleTime=1
  cfblk5 : Sum
  cfblk6 : MinMax  Inputs=3
  cfblk7 : Signum
  cfblk8 : Gain  Gain=[-203246058.316700]
  cfblk9 : UnaryMinus
  cfblk2 : Outport
  wires:
  cfblk11/1 -> cfblk5/1, cfblk10/2
  cfblk12/1 -> cfblk9/1
  cfblk3/1 -> cfblk8/1
  cfblk10/1 -> cfblk2/1
  cfblk4/1 -> cfblk3/1
  cfblk1/1 -> cfblk6/1, cfblk5/2
  cfblk5/1 -> cfblk6/2, cfblk10/1
  cfblk7/1 -> cfblk4/1
  cfblk6/1 -> cfblk4/2
  cfblk9/1 -> cfblk7/1, cfblk6/3
  cfblk8/1 -> cfblk13/1
  cfblk13/1 -> cfblk3/2

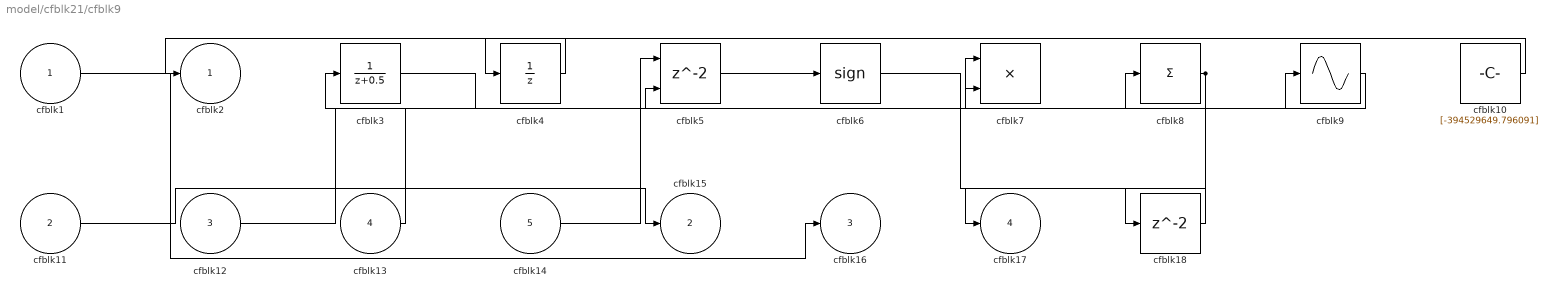
== system model/cfblk21/cfblk9 ==
  cfblk1 : Inport
  cfblk11 : Inport  Port=2
  cfblk12 : Inport  Port=3
  cfblk13 : Inport  Port=4
  cfblk14 : Inport  Port=5
  cfblk10 : Constant  Value=[-394529649.796091]  SampleTime=1
  cfblk18 : Delay  SampleTime=1
  cfblk3 : DiscreteTransferFcn  SampleTime=1
  cfblk4 : UnitDelay  HasFrameUpgradeWarning=on
  cfblk5 : Delay  ShowEnablePort=on  SampleTime=1
      settings: InputPortMap=u0,e6
  cfblk6 : Signum
  cfblk7 : Product
  cfblk8 : Sum  Inputs=+
  cfblk9 : Sin  TimeSource=Use external signal  SampleTime=0
  cfblk2 : Outport
  cfblk15 : Outport  Port=2
  cfblk16 : Outport  Port=3
  cfblk17 : Outport  Port=4
  wires:
  cfblk10/1 -> cfblk4/1
  cfblk13/1 -> cfblk3/1
  cfblk3/1 -> cfblk8/1
  cfblk8/1 -> cfblk17/1, cfblk7/2
  cfblk1/1 -> cfblk16/1
  cfblk5/1 -> cfblk6/1
  cfblk11/1 -> cfblk15/1
  cfblk9/1 -> cfblk5/2
  cfblk4/1 -> cfblk2/1
  cfblk12/1 -> cfblk9/1
  cfblk14/1 -> cfblk7/1
  cfblk6/1 -> cfblk18/1
  cfblk18/1 -> cfblk5/1

== system model/cfblk22/cfblk4 ==
  cfblk1 : Inport
  cfblk13 : Inport  Port=2
  cfblk14 : Inport  Port=3
  cfblk15 : Inport  Port=4
  cfblk16 : Inport  Port=5
  cfblk10 : Rounding
  cfblk11 : Constant  Value=[648507190.837656]  SampleTime=1
  cfblk12 : Constant  Value=[-274924446.535899]  SampleTime=1
  cfblk3 : simulink/Discrete/Transfer Fcn First Order  PoleZ=0.95  ICPrevOutput=0.0  DoSatur=off
  cfblk4 : simulink/Discrete/Transfer Fcn Lead or Lag  PoleZ=0.95  ZeroZ=0.75  ICPrevOutput=0.0  ICPrevInput=0.0  DoSatur=off
  cfblk5 : DiscreteFilter  SampleTime=1
  cfblk6 : simulink/Discrete/Difference  ICPrevInput=0.0  OutMin=[]  OutMax=[]  OutDataTypeStr=Inherit: Inherit via back propagation  OutDataType=fixdt(1, 16)  OutScaling=2^-10  DoSatur=off
  cfblk7 : DiscreteTransferFcn  SampleTime=1
  cfblk8 : Sqrt  Operator=rSqrt  AlgorithmType=Newton-Raphson
  cfblk9 : Squeeze
  cfblk2 : Outport
  cfblk17 : Outport  Port=2
  wires:
  cfblk11/1 -> cfblk7/1
  cfblk15/1 -> cfblk8/1
  cfblk16/1 -> cfblk9/1
  cfblk1/1 -> cfblk2/1
  cfblk9/1 -> cfblk10/1
  cfblk14/1 -> cfblk5/1
  cfblk3/1 -> cfblk17/1
  cfblk13/1 -> cfblk3/1
  cfblk10/1 -> cfblk4/1
  cfblk7/1 -> cfblk6/1

== system model/cfblk22/cfblk5 ==
  cfblk1 : Inport
  cfblk11 : Inport  Port=2
  cfblk12 : Inport  Port=3
  cfblk13 : Inport  Port=4
  cfblk14 : Inport  Port=5
  cfblk10 : Constant  Value=[975173899.107865]  SampleTime=1
  cfblk3 : Delay  SampleTime=1
  cfblk4 : DiscreteTransferFcn  SampleTime=1
  cfblk5 : simulink/Discrete/Tapped Delay  vinit=0.0  samptime=-1  NumDelays=1  DelayOrder=Oldest  includeCurrent=off
  cfblk6 : UnaryMinus
  cfblk7 : Assignment  DiagnosticForDimensions=Warning  IndexOptions=Index vector (dialog)  Indices=1  OutputSizes=1
  cfblk8 : Math  Operator=10^u
  cfblk9 : simulink/Math Operations/MinMax Running Resettable  Function=min  vinit=0.0
  cfblk2 : Outport
  cfblk15 : Outport  Port=2
  cfblk16 : Outport  Port=3
  wires:
  cfblk7/1 -> cfblk15/1
  cfblk11/1 -> cfblk8/1
  cfblk8/1 -> cfblk3/1
  cfblk1/1 -> cfblk5/1
  cfblk9/1 -> cfblk6/1
  cfblk12/1 -> cfblk7/1
  cfblk13/1 -> cfblk9/1
  cfblk10/1 -> cfblk9/2
  cfblk6/1 -> cfblk7/2
  cfblk3/1 -> cfblk4/1
  cfblk14/1 -> cfblk2/1
  cfblk5/1 -> cfblk16/1

== system model/cfblk22/cfblk6 ==
  cfblk1 : Inport
  cfblk6 : Inport  Port=2
  cfblk7 : Inport  Port=3
  cfblk8 : Inport  Port=4
  cfblk3 : simulink/Discrete/Transfer Fcn First Order  PoleZ=0.95  ICPrevOutput=0.0  DoSatur=off
  cfblk4 : Bias  Bias=[472249553.101924]  SaturateOnIntegerOverflow=off
  cfblk5 : PermuteDimensions
  cfblk2 : Outport
  cfblk9 : Outport  Port=2
  wires:
  cfblk4/1 -> cfblk3/1
  cfblk1/1 -> cfblk5/1
  cfblk3/1 -> cfblk2/1
  cfblk7/1 -> cfblk9/1
  cfblk5/1 -> cfblk4/1

== system model/cfblk22/cfblk7 ==
  cfblk1 : Inport
  cfblk9 : Inport  Port=2
  cfblk3 : simulink/Discrete/Tapped Delay  vinit=0.0  samptime=-1  NumDelays=1  DelayOrder=Oldest  includeCurrent=off
  cfblk4 : UnitDelay  HasFrameUpgradeWarning=on
  cfblk5 : Product
  cfblk6 : Trigonometry
  cfblk7 : Sum  Inputs=+
  cfblk8 : Math  Operator=log
  cfblk2 : Outport
  cfblk10 : Outport  Port=2
  cfblk11 : Outport  Port=3
  wires:
  cfblk3/1 -> cfblk5/1
  cfblk6/1 -> cfblk10/1
  cfblk9/1 -> cfblk7/1
  cfblk5/1 -> cfblk11/1, cfblk8/1
  cfblk7/1 -> cfblk4/1
  cfblk4/1 -> cfblk5/2
  cfblk1/1 -> cfblk3/1
  cfblk8/1 -> cfblk6/1, cfblk2/1

== system model/cfblk22/cfblk8 ==
  cfblk1 : Inport
  cfblk12 : Delay  SampleTime=1
  cfblk13 : Delay  SampleTime=1
  cfblk3 : DiscreteFilter  SampleTime=1
  cfblk4 : Delay  ShowEnablePort=on  SampleTime=1
      settings: InputPortMap=u0,e6
  cfblk5 : Delay  DelayLengthSource=Input port  SampleTime=1
      settings: InputPortMap=u0,p1
  cfblk6 : DiscreteFir  SampleTime=1
  cfblk7 : Bias  Bias=[39582363.719997]  SaturateOnIntegerOverflow=off
  cfblk8 : Abs  SaturateOnIntegerOverflow=off
  cfblk9 : Constant  Value=[-572467626.401414]  SampleTime=1
  cfblk2 : Outport
  cfblk10 : Outport  Port=2
  cfblk11 : Outport  Port=3
  wires:
  cfblk7/1 -> cfblk10/1
  cfblk8/1 -> cfblk11/1, cfblk5/2
  cfblk3/1 -> cfblk8/1
  cfblk4/1 -> cfblk6/1
  cfblk1/1 -> cfblk4/1
  cfblk9/1 -> cfblk2/1, cfblk5/1, cfblk7/1
  cfblk6/1 -> cfblk12/1
  cfblk12/1 -> cfblk4/2
  cfblk5/1 -> cfblk13/1
  cfblk13/1 -> cfblk3/1

== system model/cfblk23/cfblk5 ==
  cfblk1 : Inport
  cfblk6 : Inport  Port=2
  cfblk7 : Inport  Port=3
  cfblk8 : Inport  Port=4
  cfblk3 : Squeeze
  cfblk4 : PermuteDimensions
  cfblk5 : Constant  Value=[643765402.773875]  SampleTime=1
  cfblk2 : Outport
  wires:
  cfblk5/1 -> cfblk2/1
  cfblk8/1 -> cfblk4/1
  cfblk1/1 -> cfblk3/1

== system model/cfblk23/cfblk6 ==
  cfblk1 : Inport
  cfblk8 : Inport  Port=2
  cfblk9 : Inport  Port=3
  cfblk11 : Delay  SampleTime=1
  cfblk3 : simulink/Discrete/Difference  ICPrevInput=0.0  OutMin=[]  OutMax=[]  OutDataTypeStr=Inherit: Inherit via back propagation  OutDataType=fixdt(1, 16)  OutScaling=2^-10  DoSatur=off
  cfblk4 : Delay  SampleTime=1
  cfblk5 : Delay  ShowEnablePort=on  SampleTime=1
      settings: InputPortMap=u0,e6
  cfblk6 : Math  Operator=log
  cfblk7 : Assignment  DiagnosticForDimensions=Warning  IndexOptions=Index vector (dialog)  Indices=1  OutputSizes=1
  cfblk2 : Outport
  cfblk10 : Outport  Port=2
  wires:
  cfblk5/1 -> cfblk10/1
  cfblk4/1 -> cfblk6/1
  cfblk6/1 -> cfblk5/1, cfblk11/1
  cfblk3/1 -> cfblk7/1
  cfblk9/1 -> cfblk7/2
  cfblk1/1 -> cfblk2/1
  cfblk7/1 -> cfblk4/1
  cfblk8/1 -> cfblk5/2
  cfblk11/1 -> cfblk3/1

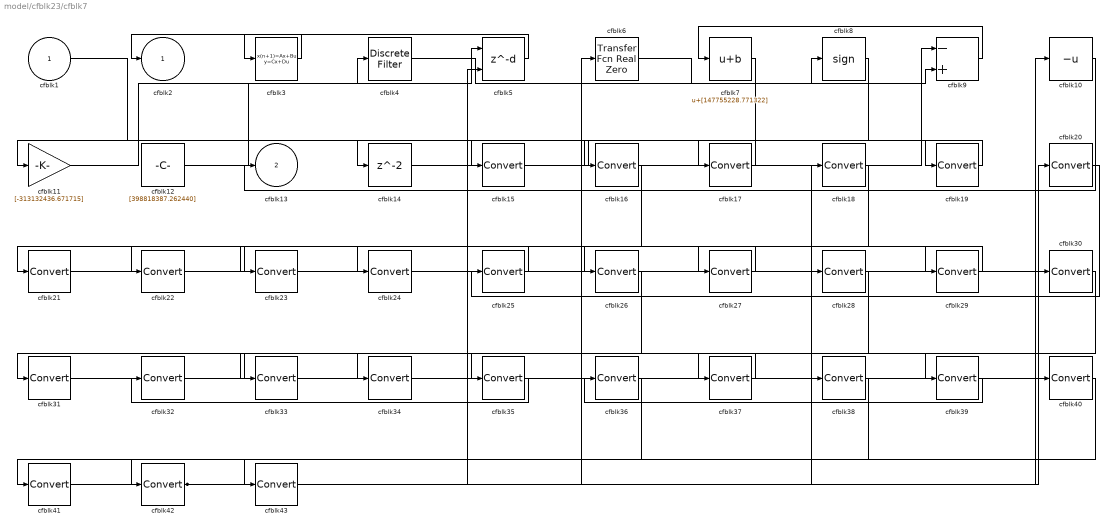
== system model/cfblk23/cfblk7 ==
  cfblk1 : Inport
  cfblk10 : UnaryMinus
  cfblk11 : Gain  Gain=[-313132436.671715]
  cfblk12 : Constant  Value=[398818387.262440]  SampleTime=1
  cfblk14 : Delay  SampleTime=1
  cfblk{15..43} (29 alike) : DataTypeConversion  SaturateOnIntegerOverflow=off  RndMeth=Floor
  cfblk3 : DiscreteStateSpace
  cfblk4 : DiscreteFilter  SampleTime=1
  cfblk5 : Delay  DelayLengthSource=Input port  SampleTime=1
      settings: InputPortMap=u0,p1
  cfblk6 : simulink/Discrete/Transfer Fcn Real Zero  ZeroZ=0.75  ICPrevInput=0.0  DoSatur=off
  cfblk7 : Bias  Bias=[147755228.771322]  SaturateOnIntegerOverflow=off
  cfblk8 : Signum
  cfblk9 : Sum  Inputs=-+
  cfblk2 : Outport
  cfblk13 : Outport  Port=2
  wires:
  cfblk8/1 -> cfblk11/1
  cfblk11/1 -> cfblk5/1
  cfblk9/1 -> cfblk7/1
  cfblk5/1 -> cfblk3/1
  cfblk6/1 -> cfblk8/1
  cfblk12/1 -> cfblk4/1
  cfblk3/1 -> cfblk2/1
  cfblk10/1 -> cfblk13/1
  cfblk4/1 -> cfblk9/2
  cfblk7/1 -> cfblk14/1
  cfblk14/1 -> cfblk9/1
  cfblk1/1 -> cfblk17/1
  cfblk17/1 -> cfblk15/1
  cfblk15/1 -> cfblk19/1
  cfblk19/1 -> cfblk16/1
  cfblk16/1 -> cfblk21/1
  cfblk21/1 -> cfblk18/1
  cfblk18/1 -> cfblk23/1
  cfblk23/1 -> cfblk20/1
  cfblk20/1 -> cfblk25/1
  cfblk25/1 -> cfblk22/1
  cfblk22/1 -> cfblk27/1
  cfblk27/1 -> cfblk24/1
  cfblk24/1 -> cfblk29/1
  cfblk29/1 -> cfblk26/1
  cfblk26/1 -> cfblk31/1
  cfblk31/1 -> cfblk28/1
  cfblk28/1 -> cfblk33/1
  cfblk33/1 -> cfblk30/1
  cfblk30/1 -> cfblk35/1
  cfblk35/1 -> cfblk32/1
  cfblk32/1 -> cfblk37/1
  cfblk37/1 -> cfblk34/1
  cfblk34/1 -> cfblk39/1
  cfblk39/1 -> cfblk36/1
  cfblk40/1 -> cfblk42/1
  cfblk36/1 -> cfblk41/1
  cfblk41/1 -> cfblk38/1
  cfblk42/1 -> cfblk5/2, cfblk10/1, cfblk6/1
  cfblk38/1 -> cfblk43/1
  cfblk43/1 -> cfblk40/1

== system model/cfblk25/cfblk9 ==
  cfblk1 : Inport
  cfblk5 : Inport  Port=2
  cfblk6 : Inport  Port=3
  cfblk3 : Product  Inputs=*
  cfblk4 : Constant  Value=[-224110532.540288]  SampleTime=1
  cfblk2 : Outport
  cfblk7 : Outport  Port=2
  wires:
  cfblk1/1 -> cfblk7/1
  cfblk4/1 -> cfblk2/1
  cfblk5/1 -> cfblk3/1

== system model/cfblk26/cfblk10 ==
  cfblk1 : Inport
  cfblk10 : Inport  Port=2
  cfblk11 : Inport  Port=3
  cfblk3 : DiscreteFilter  SampleTime=1
  cfblk4 : slpidlib/PID Controller (2DOF)  Controller=PID  Form=Parallel  TimeDomain=Discrete-time  UseExternalTs=off  SampleTime=1  IntegratorMethod=Forward Euler  FilterMethod=Forward Euler  ControllerParametersSource=internal  P=1  I=1  UseKiTs=off  D=0  N=100  UseFilter=on  b=1  c=1  TunerSelectOption=Transfer Function Based (PID Tuner App)  InitialConditionSource=internal  InitialConditionForIntegrator=0  InitialConditionForFilter=0  DifferentiatorICPrevScaledInput=0  ExternalReset=none  TrackingMode=off  Kt=1  LimitOutput=off  SatLimitsSource=internal  UpperSaturationLimit=inf  LowerSaturationLimit=-inf  LinearizeAsGain=off  AntiWindupMode=none  Kb=1  LimitIntegrator=off  UpperIntegratorSaturationLimit=inf  LowerIntegratorSaturationLimit=-inf  POutMin=[]  POutMax=[]  IOutMin=[]  IOutMax=[]  DOutMin=[]  DOutMax=[]  NOutMin=[]  NOutMax=[]  bOutMin=[]  bOutMax=[]  cOutMin=[]  cOutMax=[]  SumOutMin=[]  SumOutMax=[]  SaturationOutMin=[]  SaturationOutMax=[]  PParamMin=[]  PParamMax=[]  IParamMin=[]  IParamMax=[]  DParamMin=[]  DParamMax=[]  NParamMin=[]  NParamMax=[]  bParamMin=[]  bParamMax=[]  cParamMin=[]  cParamMax=[]  KbParamMin=[]  KbParamMax=[]  KtParamMin=[]  KtParamMax=[]  KbOutMin=[]  KbOutMax=[]  KtOutMin=[]  KtOutMax=[]  IntegratorOutMin=[]  IntegratorOutMax=[]  FilterOutMin=[]  FilterOutMax=[]  SumI1OutMin=[]  SumI1OutMax=[]  SumI2OutMin=[]  SumI2OutMax=[]  SumI3OutMin=[]  SumI3OutMax=[]  SumI4OutMin=[]  SumI4OutMax=[]  SumDOutMin=[]  SumDOutMax=[]  Sum1OutMin=[]  Sum1OutMax=[]  Sum2OutMin=[]  Sum2OutMax=[]  Sum3OutMin=[]  Sum3OutMax=[]  DifferentiatorOutMin=[]  DifferentiatorOutMax=[]  FilterDiffOutCoefMin=[]  FilterDiffOutCoefMax=[]  ReciprocalOutMin=[]  ReciprocalOutMax=[]  SumDenOutMin=[]  SumDenOutMax=[]  SumNumOutMin=[]  SumNumOutMax=[]  DivideOutMin=[]  DivideOutMax=[]  UdiffTsProdOutMin=[]  UdiffTsProdOutMax=[]  NTsProdOutMin=[]  NTsProdOutMax=[]  UintegralTsProdOutMin=[]  UintegralTsProdOutMax=[]  UngainTsProdOutMin=[]  UngainTsProdOutMax=[]  ClampingZeroOutDataTypeStr=Inherit: Inherit via back propagation  ClampingZeroOutMin=[]  ClampingZeroOutMax=[]  FilterDenConstantOutDataTypeStr=Inherit: Inherit via back propagation  FilterDenConstantOutMin=[]  FilterDenConstantOutMax=[]  PCopyOutDataTypeStr=Inherit: Inherit via back propagation  PCopyOutMin=[]  PCopyOutMax=[]  NCopyOutDataTypeStr=Inherit: Inherit via back propagation  NCopyOutMin=[]  NCopyOutMax=[]  IntegratorContinuousStateAttributes=''  IntegratorStateMustResolveToSignalObject=off  IntegratorRTWStateStorageClass=Auto  FilterContinuousStateAttributes=''  FilterStateMustResolveToSignalObject=off  FilterRTWStateStorageClass=Auto  ParallelPVariant=InternalParameters  IdealPVariant=Disabled  IVariant=InternalParameters  DVariant=InternalParameters  bVariant=InternalParameters  cVariant=InternalParameters  IntegratorVariant=Discrete  SatVariant=Disabled  AWVariant=Passthrough  PCopyVariant=Disabled  TRVariant=Disabled  FdbkBlocksVariant=Forward  IdealPFdbkVariant=Disabled  SatFdbkVariant=Disabled  DerivativeFilterVariant=ForwardEulerFilter  NVariant=InternalParameters  NCopyVariant=Disabled  FilterICVariant=InternalICsFilter  IntegratorICVariant=InternalICs  ExternalResetVariant=Disabled  TRSumVariant=Passthrough  SumFdbkVariant=Disabled  SumVariant=Sum_PID  TsampFilterVariant=InternalTs  TsampNgainVariant=Passthrough  TsampIntegralVariant=Disabled_SignalSpec  ExternalSaturationOutDataTypeStr=Inherit: Same as second input
      settings: LibrarySourceBlock=simulink/Discrete/Discrete PID Controller (2DOF)
  cfblk5 : Product
  cfblk6 : MinMax  Function=max
  cfblk7 : Reshape
  cfblk8 : Constant  Value=[-444285898.107445]  SampleTime=1
  cfblk9 : Constant  Value=[110561584.175398]  SampleTime=1
  cfblk2 : Outport
  cfblk12 : Outport  Port=2
  wires:
  cfblk9/1 -> cfblk3/1
  cfblk11/1 -> cfblk6/1
  cfblk7/1 -> cfblk4/1
  cfblk1/1 -> cfblk7/1
  cfblk10/1 -> cfblk12/1
  cfblk8/1 -> cfblk4/2
  cfblk5/1 -> cfblk2/1
  cfblk4/1 -> cfblk5/1
  cfblk6/1 -> cfblk5/2
